simulink model "tamami"  (R2020a)
settings: Solver=VariableStepAuto  StartTime=0.0  StopTime=10.0  RelTol=1e-3
undefined symbols (not defined in the file): b, g, I, l, M, m, sigbuilder_block
libraries: simulink x1, simulink_extras x1, vrlib x1
settings Model: Creator=Esra  LastModifiedBy=Esra

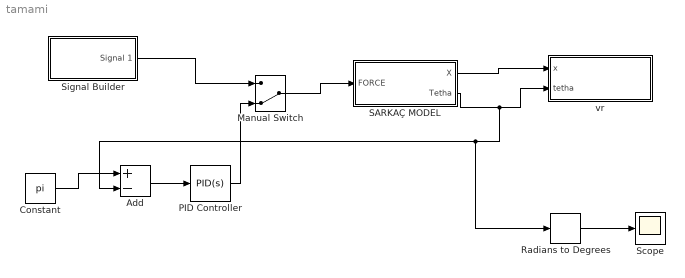
== system tamami ==
  Add : Sum  Inputs=+-
  Constant : Constant  Value=pi
  Manual Switch : ManualSwitch  CurrentSetting=0
  PID Controller : simulink/Continuous/PID Controller  Controller=PID  Form=Parallel  TimeDomain=Continuous-time  UseExternalTs=off  SampleTime=-1  IntegratorMethod=Forward Euler  FilterMethod=Forward Euler  ControllerParametersSource=internal  P=1000  I=1  D=200  UseFilter=on  N=100  TunerSelectOption=Transfer Function Based (PID Tuner App)  InitialConditionSource=internal  InitialConditionForIntegrator=0  InitialConditionForFilter=0  DifferentiatorICPrevScaledInput=0  ExternalReset=none  TrackingMode=off  Kt=1  LimitOutput=off  UpperSaturationLimit=inf  LowerSaturationLimit=-inf  LinearizeAsGain=on  AntiWindupMode=none  Kb=1  POutMin=[]  POutMax=[]  IOutMin=[]  IOutMax=[]  DOutMin=[]  DOutMax=[]  NOutMin=[]  NOutMax=[]  SumOutMin=[]  SumOutMax=[]  SaturationOutMin=[]  SaturationOutMax=[]  PParamMin=[]  PParamMax=[]  IParamMin=[]  IParamMax=[]  DParamMin=[]  DParamMax=[]  NParamMin=[]  NParamMax=[]  KbParamMin=[]  KbParamMax=[]  KtParamMin=[]  KtParamMax=[]  KbOutMin=[]  KbOutMax=[]  KtOutMin=[]  KtOutMax=[]  IntegratorOutMin=[]  IntegratorOutMax=[]  FilterOutMin=[]  FilterOutMax=[]  SumI1OutMin=[]  SumI1OutMax=[]  SumI2OutMin=[]  SumI2OutMax=[]  SumI3OutMin=[]  SumI3OutMax=[]  SumI4OutMin=[]  SumI4OutMax=[]  SumDOutMin=[]  SumDOutMax=[]  DifferentiatorOutMin=[]  DifferentiatorOutMax=[]  FilterDiffOutCoefMin=[]  FilterDiffOutCoefMax=[]  ReciprocalOutMin=[]  ReciprocalOutMax=[]  SumDenOutMin=[]  SumDenOutMax=[]  SumNumOutMin=[]  SumNumOutMax=[]  DivideOutMin=[]  DivideOutMax=[]  UdiffTsProdOutMin=[]  UdiffTsProdOutMax=[]  NTsProdOutMin=[]  NTsProdOutMax=[]  UintegralTsProdOutMin=[]  UintegralTsProdOutMax=[]  UngainTsProdOutMin=[]  UngainTsProdOutMax=[]  IntegratorContinuousStateAttributes=''  IntegratorStateMustResolveToSignalObject=off  IntegratorRTWStateStorageClass=Auto  FilterContinuousStateAttributes=''  FilterStateMustResolveToSignalObject=off  FilterRTWStateStorageClass=Auto  ParallelPVariant=InternalParameters  IdealPVariant=Disabled  IVariant=InternalParameters  DVariant=InternalParameters  IntegratorVariant=Continuous  SatVariant=Disabled  AWVariant=Passthrough  PCopyVariant=Disabled  TRVariant=Disabled  FdbkBlocksVariant=Forward  IdealPFdbkVariant=Disabled  SatFdbkVariant=Disabled  DerivativeFilterVariant=ContFilter  NVariant=InternalParameters  NCopyVariant=Disabled  FilterICVariant=InternalICsFilter  IntegratorICVariant=InternalICs  ExternalResetVariant=Disabled  TRSumVariant=Passthrough  SumFdbkVariant=Disabled  SumVariant=Sum_PID  TsampFilterVariant=InternalTs  TsampNgainVariant=Passthrough  TsampIntegralVariant=Passthrough
  Radians to Degrees : simulink_extras/Transformations/Radians to Degrees
  SARKAÇ MODEL : Subsystem
  Scope : Scope
  Signal Builder : Subsystem  Tag=STV Subsys  LoadFcn=sigbuilder_block('load');  StartFcn=sigbuilder_block('start');  StopFcn=sigbuilder_block('stop');  ClipboardFcn=sigbuilder_block('clipboard');  mask(Sigbuilder block){tuvar=[0:10]}
      mask help: Simulink:masks:SigbuilderBlock_MD
      mask init:
      | if ~strcmp(get_param(bdroot(gcbh),'SimulationStatus'),'stopped') tuvar = sigbuilder_block('maskInit'); end
      settings: CopyFcn=sigbuilder_block('copy');  DeleteFcn=sigbuilder_block('delete');  ModelCloseFcn=sigbuilder_block('modelClose');  PreSaveFcn=sigbuilder_block('preSave');  PauseFcn=sigbuilder_block('pause');  ContinueFcn=sigbuilder_block('continue');  NameChangeFcn=sigbuilder_block('namechange');  OpenFcn=sigbuilder_block('open',[437.6 153 550.4 359.25 ]);  CloseFcn=sigbuilder_block('close');
      mask Display: plot(0, 0, 100, 100,[2, 2, 32, 32, 2], [68, 8, 8, 68, 68],[32, 2], [38, 38], [32, 19, 2],[53, 60, 44], [32, 17, 17, 2],[16, 16, 31, 31]);txt = getActiveGroup(gcbh);text(2, 100, txt,'verticalAlignment', 'top');
  vr : Subsystem
  wires:
  SARKAÇ MODEL/1(X) -> vr/1(x)
  SARKAÇ MODEL/2(Tetha) -> Radians to Degrees/1, Add/2, vr/2(tetha)
  Constant/1 -> Add/1
  Add/1 -> PID Controller/1
  PID Controller/1 -> Manual Switch/2
  Signal Builder/1(Signal 1) -> Manual Switch/1
  Manual Switch/1 -> SARKAÇ MODEL/1(FORCE)
  Radians to Degrees/1 -> Scope/1

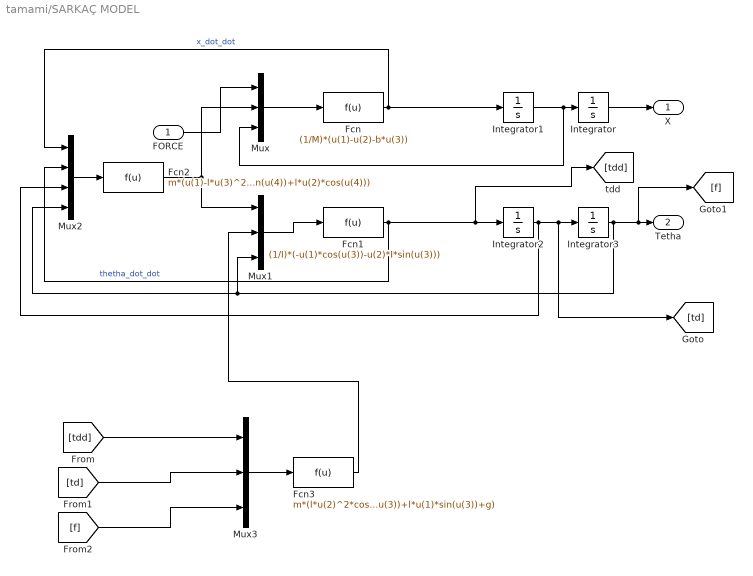
== system tamami/SARKAÇ MODEL ==
  FORCE : Inport
  Fcn : Fcn  Expr=(1/M)*(u(1)-u(2)-b*u(3))
  Fcn1 : Fcn  Expr=(1/I)*(-u(1)*cos(u(3))-u(2)*I*sin(u(3)))
  Fcn2 : Fcn  Expr=m*(u(1)-l*u(3)^2*sin(u(4))+l*u(2)*cos(u(4)))
  Fcn3 : Fcn  Expr=m*(l*u(2)^2*cos(u(3))+l*u(1)*sin(u(3))+g)
  Integrator : Integrator
  Integrator1 : Integrator
  Integrator2 : Integrator
  Integrator3 : Integrator  InitialCondition=pi-0.1
  Mux : Mux  Inputs=3
  Mux1 : Mux  Inputs=3
  Mux2 : Mux
  Mux3 : Mux  Inputs=3
  X : Outport
  Tetha : Outport  Port=2
  wires:
  Integrator1/1 -> Mux/3, Integrator/1
  Fcn/1 -> Mux2/1, Integrator1/1  "x_dot_dot"
  Fcn1/1 -> Mux2/2, [tdd], Integrator2/1  "thetha_dot_dot"
  FORCE/1 -> Mux/1
  Fcn2/1 -> Mux1/1, Mux/2
  Mux/1 -> Fcn/1
  Integrator/1 -> X/1
  Mux1/1 -> Fcn1/1
  Fcn3/1 -> Mux1/2
  Integrator2/1 -> Mux2/3, [td], Integrator3/1
  Integrator3/1 -> Mux1/3, Mux2/4, [f], Tetha/1
  Mux2/1 -> Fcn2/1
  [tdd] -> Mux3/1
  [td] -> Mux3/2
  [f] -> Mux3/3
  Mux3/1 -> Fcn3/1

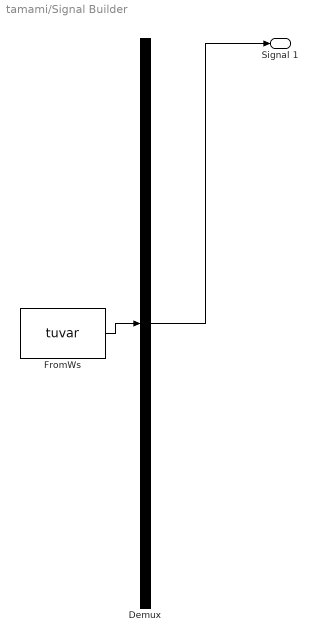
== system tamami/Signal Builder ==
  Demux : Demux  Tag=STV Demux  Outputs=1
      settings: DisplayOption=none
  FromWs : FromWorkspace  Tag=STV FromWs  VariableName=tuvar
      SigBuilderData=|
      | common.afterFinalStr = 'Extrapolate'
      | common.sampleTime = 0
      | dataSet.timeRange = [0 10]
      | dataSet.name = 'Group 1'
      | sbobj.Groups.Name = 'Group 1'
      | sbobj.Groups.Signals.Name = 'Signal 1'
      | sbobj.Groups.Signals.XData = [0 0.96 0.96 2.02 2.02 10]
      | sbobj.Groups.Signals.YData = [0 0 4.82 4.82 0 0]
  Signal 1 : Outport  Tag=STV Outport
  wires:
  Demux/1 -> Signal 1/1
  FromWs/1 -> Demux/1

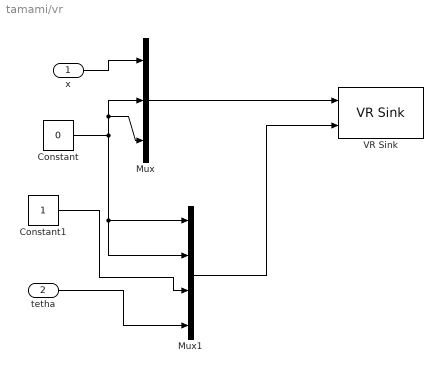
== system tamami/vr ==
  x : Inport
  tetha : Inport  Port=2
  Constant : Constant  Value=0
  Constant1 : Constant
  Mux : Mux  Inputs=3
  Mux1 : Mux
  VR Sink : vrlib/VR Sink  InstantiateOnLoad=on  SampleTime=0.0001  ViewEnable=on  RemoteChange=off  RemoteView=off  FieldsWritten=Araba.translation.3.1.1.double#Mentese2.rotation.4.1.1.double  WorldFileName=vrml1.wrl  AutoView=off  VideoDimensions=[]  AllowVariableSize=off
  wires:
  x/1 -> Mux/1
  Constant/1 -> Mux/2, Mux/3, Mux1/1, Mux1/2
  Mux/1 -> VR Sink/1
  tetha/1 -> Mux1/4
  Constant1/1 -> Mux1/3
  Mux1/1 -> VR Sink/2
